simulink model "model_observer_test"  (R2013b)
settings: Solver=ode45  StartTime=0.0  StopTime=10.0  FixedStep=0.2  RelTol=1e-3
values from neighbouring files (symbols this model uses):
  A = A-B*K    [variables.m]
  B = B    [variables.m]
  C = C    [variables.m]
  K = acker(A, B, K_poles)    [variables.m]
  L = acker(A', C', L_poles)    [variables.m]
settings Model: Creator=Sander  LastModifiedBy=Sander

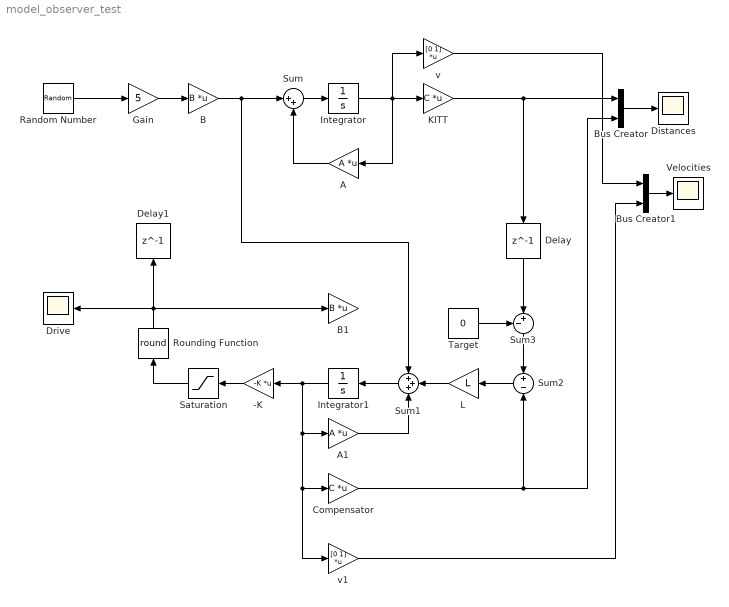
== system model_observer_test ==
  -K : Gain  Gain=-K  Multiplication=Matrix(K*u)
  A : Gain  Gain=A  Multiplication=Matrix(K*u)
  A1 : Gain  Gain=A  Multiplication=Matrix(K*u)
  B : Gain  Gain=B  Multiplication=Matrix(K*u)
  B1 : Gain  Gain=B  Multiplication=Matrix(K*u)
  Bus Creator : BusCreator  Inputs=2
  Bus Creator1 : BusCreator  Inputs=2
  Compensator : Gain  Gain=C  Multiplication=Matrix(K*u)
  Delay : Delay  DelayLength=1  InitialCondition=300  SampleTime=0.05
  Delay1 : Delay  DelayLength=1  InitialCondition=0  SampleTime=0.05
  Distances : Scope
      settings: ShowLegends=on  TimeRange=8.13238770685579  YMin=27.18749999999995  YMax=115.3125  SaveName=distances
  Drive : Scope
      settings: ShowLegends=on  SaveName=drive
  Gain : Gain  Gain=5
  Integrator : Integrator  InitialCondition=[300;5]
  Integrator1 : Integrator  InitialCondition=[294;0]
  KITT : Gain  Gain=C  Multiplication=Matrix(K*u)
  L : Gain  Gain=L
  Random Number : RandomNumber  Variance=0.05  SampleTime=0.1
  Rounding Function : Rounding  Operator=round
  Saturation : Saturate  UpperLimit=10  LowerLimit=-10  RndMeth=Round
      settings: LockScale=on
  Sum : Sum  Inputs=|++
  Sum1 : Sum  Inputs=+++
  Sum2 : Sum  Inputs=+|-
  Sum3 : Sum  Inputs=-+|
  Target : Constant  Value=0
  Velocities : Scope
      settings: ShowLegends=on  TimeRange=8.13238770685579  YMin=27.18749999999995  YMax=115.3125  SaveName=distances1
  v : Gain  Gain=[0 1]  Multiplication=Matrix(K*u)
  v1 : Gain  Gain=[0 1]  Multiplication=Matrix(K*u)
  wires:
  A/1 -> Sum/2
  Sum/1 -> Integrator/1
  Integrator/1 -> v/1, KITT/1, A/1
  Sum1/1 -> Integrator1/1
  A1/1 -> Sum1/3
  L/1 -> Sum1/2
  Sum2/1 -> L/1
  Bus Creator/1 -> Distances/1
  Compensator/1 -> Bus Creator/2, Sum2/2
  KITT/1 -> Delay/1, Bus Creator/1
  -K/1 -> Saturation/1
  Sum3/1 -> Sum2/1
  Target/1 -> Sum3/1
  Rounding Function/1 -> Drive/1, Delay1/1, B1/1
  Saturation/1 -> Rounding Function/1
  Delay/1 -> Sum3/2
  Integrator1/1 -> -K/1, v1/1, Compensator/1, A1/1
  Bus Creator1/1 -> Velocities/1
  v1/1 -> Bus Creator1/2
  v/1 -> Bus Creator1/1
  Random Number/1 -> Gain/1
  Gain/1 -> B/1
  B/1 -> Sum1/1, Sum/1
